simulink model "ReactorDistillation_scenario2_ratioV"  (R2024a)
settings: Solver=VariableStepAuto  StartTime=0.0  StopTime=1200  RelTol=1e-3
libraries: slpidlib x4
settings Model: Creator=tmlouw  LastModifiedBy=tmlouw

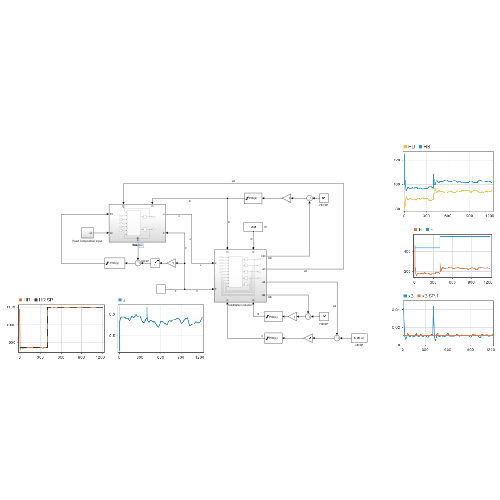
[thumbnail: Simulink's stored preview of the top-level diagram]
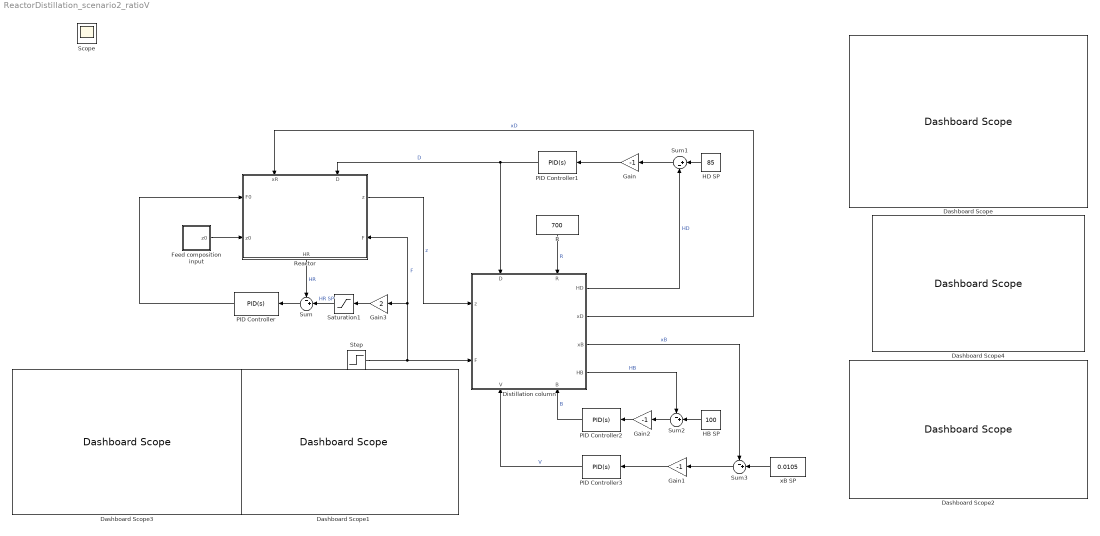
== system ReactorDistillation_scenario2_ratioV ==
  Dashboard Scope{,1,3..4} (4 alike) : DashboardScope
  Dashboard Scope2 : DashboardScope  Ymin=0  Ymax=0.05  ScaleAtStop=off
  Distillation column : Subsystem
      settings: PortSchema="{\"entries\":[{\"content\":{\"sides\":[{\"content\":{\"connectorIds\":[\"In1\",\"In2\"]},\"type\":\"ConnectorPlacement.EquallySpacedRectSide\",\"uuid\":\"ab420837-8800-483a-94a8-8143737a47c2\"},{\"content\":{\"connectorIds\":[\"Out1\",\"Out2\",\"Out3\",\"Out4\"],\"side\":\"RIGHT\"},\"type\":\"ConnectorPlacement.EquallySpacedRectSide\",\"uuid\":\"9920b73b-e391-416a-a827-f17b334a8e6d\"},{\"content\":{\"connectorIds\":[\"In3\",\"In4\"],\"side\":\"TOP\"},\"type\":\"ConnectorPlacement.EquallySpacedRectSide\",\"uuid\":\"f76ae38a-6a7c-4206-be40-6de8ba6ae5dc\"},{\"content\":{\"connectorIds\":[\"In5\",\"In6\"],\"side\":\"BOTTOM\"},\"type\":\"ConnectorPlacement.EquallySpacedRectSide\",\"uuid\":\"fa4d76dd-125e-48cb-976d-db25120835fd\"}]},\"type\":\"ConnectorPlacement.EquallySpacedConnector\",\"uuid\":\"aba5cf7b-c109-4372-afa3-985106281a24\"}],\"packageUris\":[\"http://schema.mathworks.com/mf0/Connector/R2020b\"],\"version\":\"1.0\"}"
  Feed composition input : Subsystem
  Gain : Gain  Gain=-1
  Gain1 : Gain  Gain=-1
  Gain2 : Gain  Gain=-1
  Gain3 : Gain  Gain=2
  HB SP : Constant  Value=100
  HD SP : Constant  Value=85
  PID Controller : slpidlib/PID Controller  Controller=PID  Form=Parallel  TimeDomain=Continuous-time  UseExternalTs=off  SampleTime=-1  IntegratorMethod=Forward Euler  FilterMethod=Forward Euler  ControllerParametersSource=internal  P=10  I=1  UseKiTs=off  D=0  UseExternalDerivativeSource=off  N=100  UseFilter=on  TunerSelectOption=Transfer Function Based (PID Tuner App)  InitialConditionSource=internal  InitialConditionForIntegrator=210  InitialConditionForFilter=0  DifferentiatorICPrevScaledInput=0  ExternalReset=none  TrackingMode=off  Kt=1  LimitOutput=on  SatLimitsSource=internal  UpperSaturationLimit=inf  LowerSaturationLimit=0  LinearizeAsGain=on  AntiWindupMode=none  Kb=1  LimitIntegrator=off  UpperIntegratorSaturationLimit=inf  LowerIntegratorSaturationLimit=-inf  POutMin=[]  POutMax=[]  IOutMin=[]  IOutMax=[]  DOutMin=[]  DOutMax=[]  NOutMin=[]  NOutMax=[]  SumOutMin=[]  SumOutMax=[]  SaturationOutMin=[]  SaturationOutMax=[]  PParamMin=[]  PParamMax=[]  IParamMin=[]  IParamMax=[]  DParamMin=[]  DParamMax=[]  NParamMin=[]  NParamMax=[]  KbParamMin=[]  KbParamMax=[]  KtParamMin=[]  KtParamMax=[]  KbOutMin=[]  KbOutMax=[]  KtOutMin=[]  KtOutMax=[]  IntegratorOutMin=[]  IntegratorOutMax=[]  FilterOutMin=[]  FilterOutMax=[]  SumI1OutMin=[]  SumI1OutMax=[]  SumI2OutMin=[]  SumI2OutMax=[]  SumI3OutMin=[]  SumI3OutMax=[]  SumI4OutMin=[]  SumI4OutMax=[]  SumDOutMin=[]  SumDOutMax=[]  DifferentiatorOutMin=[]  DifferentiatorOutMax=[]  FilterDiffOutCoefMin=[]  FilterDiffOutCoefMax=[]  ReciprocalOutMin=[]  ReciprocalOutMax=[]  SumDenOutMin=[]  SumDenOutMax=[]  SumNumOutMin=[]  SumNumOutMax=[]  DivideOutMin=[]  DivideOutMax=[]  UdiffTsProdOutMin=[]  UdiffTsProdOutMax=[]  NTsProdOutMin=[]  NTsProdOutMax=[]  UintegralTsProdOutMin=[]  UintegralTsProdOutMax=[]  UngainTsProdOutMin=[]  UngainTsProdOutMax=[]  ClampingZeroOutDataTypeStr=Inherit: Inherit via back propagation  ClampingZeroOutMin=[]  ClampingZeroOutMax=[]  FilterDenConstantOutDataTypeStr=Inherit: Inherit via back propagation  FilterDenConstantOutMin=[]  FilterDenConstantOutMax=[]  PCopyOutDataTypeStr=Inherit: Inherit via back propagation  PCopyOutMin=[]  PCopyOutMax=[]  NCopyOutDataTypeStr=Inherit: Inherit via back propagation  NCopyOutMin=[]  NCopyOutMax=[]  IntegratorContinuousStateAttributes=''  IntegratorStateMustResolveToSignalObject=off  IntegratorRTWStateStorageClass=Auto  FilterContinuousStateAttributes=''  FilterStateMustResolveToSignalObject=off  FilterRTWStateStorageClass=Auto  ParallelPVariant=InternalParameters  IdealPVariant=Disabled  IVariant=InternalParameters  DVariant=InternalParameters  IntegratorVariant=Continuous  SatVariant=Enabled  AWVariant=Passthrough  PCopyVariant=Disabled  TRVariant=Disabled  FdbkBlocksVariant=Forward  IdealPFdbkVariant=Disabled  SatFdbkVariant=Disabled  DerivativeFilterVariant=ContFilter  NVariant=InternalParameters  NCopyVariant=Disabled  FilterICVariant=InternalICsFilter  IntegratorICVariant=InternalICs  ExternalResetVariant=Disabled  TRSumVariant=Passthrough  SumFdbkVariant=Disabled  SumVariant=Sum_PID  TsampFilterVariant=InternalTs  TsampNgainVariant=Passthrough  TsampIntegralVariant=Disabled_SignalSpec  ExternalSaturationOutDataTypeStr=Inherit: Same as second input  DerivativeSourceVariant=ErrorSignal
  PID Controller1 : slpidlib/PID Controller  Controller=PID  Form=Parallel  TimeDomain=Continuous-time  UseExternalTs=off  SampleTime=-1  IntegratorMethod=Forward Euler  FilterMethod=Forward Euler  ControllerParametersSource=internal  P=10  I=0  UseKiTs=off  D=0  UseExternalDerivativeSource=off  N=100  UseFilter=on  TunerSelectOption=Transfer Function Based (PID Tuner App)  InitialConditionSource=internal  InitialConditionForIntegrator=225  InitialConditionForFilter=0  DifferentiatorICPrevScaledInput=0  ExternalReset=none  TrackingMode=off  Kt=1  LimitOutput=on  SatLimitsSource=internal  UpperSaturationLimit=inf  LowerSaturationLimit=0  LinearizeAsGain=on  AntiWindupMode=none  Kb=1  LimitIntegrator=off  UpperIntegratorSaturationLimit=inf  LowerIntegratorSaturationLimit=-inf  POutMin=[]  POutMax=[]  IOutMin=[]  IOutMax=[]  DOutMin=[]  DOutMax=[]  NOutMin=[]  NOutMax=[]  SumOutMin=[]  SumOutMax=[]  SaturationOutMin=[]  SaturationOutMax=[]  PParamMin=[]  PParamMax=[]  IParamMin=[]  IParamMax=[]  DParamMin=[]  DParamMax=[]  NParamMin=[]  NParamMax=[]  KbParamMin=[]  KbParamMax=[]  KtParamMin=[]  KtParamMax=[]  KbOutMin=[]  KbOutMax=[]  KtOutMin=[]  KtOutMax=[]  IntegratorOutMin=[]  IntegratorOutMax=[]  FilterOutMin=[]  FilterOutMax=[]  SumI1OutMin=[]  SumI1OutMax=[]  SumI2OutMin=[]  SumI2OutMax=[]  SumI3OutMin=[]  SumI3OutMax=[]  SumI4OutMin=[]  SumI4OutMax=[]  SumDOutMin=[]  SumDOutMax=[]  DifferentiatorOutMin=[]  DifferentiatorOutMax=[]  FilterDiffOutCoefMin=[]  FilterDiffOutCoefMax=[]  ReciprocalOutMin=[]  ReciprocalOutMax=[]  SumDenOutMin=[]  SumDenOutMax=[]  SumNumOutMin=[]  SumNumOutMax=[]  DivideOutMin=[]  DivideOutMax=[]  UdiffTsProdOutMin=[]  UdiffTsProdOutMax=[]  NTsProdOutMin=[]  NTsProdOutMax=[]  UintegralTsProdOutMin=[]  UintegralTsProdOutMax=[]  UngainTsProdOutMin=[]  UngainTsProdOutMax=[]  ClampingZeroOutDataTypeStr=Inherit: Inherit via back propagation  ClampingZeroOutMin=[]  ClampingZeroOutMax=[]  FilterDenConstantOutDataTypeStr=Inherit: Inherit via back propagation  FilterDenConstantOutMin=[]  FilterDenConstantOutMax=[]  PCopyOutDataTypeStr=Inherit: Inherit via back propagation  PCopyOutMin=[]  PCopyOutMax=[]  NCopyOutDataTypeStr=Inherit: Inherit via back propagation  NCopyOutMin=[]  NCopyOutMax=[]  IntegratorContinuousStateAttributes=''  IntegratorStateMustResolveToSignalObject=off  IntegratorRTWStateStorageClass=Auto  FilterContinuousStateAttributes=''  FilterStateMustResolveToSignalObject=off  FilterRTWStateStorageClass=Auto  ParallelPVariant=InternalParameters  IdealPVariant=Disabled  IVariant=InternalParameters  DVariant=InternalParameters  IntegratorVariant=Continuous  SatVariant=Enabled  AWVariant=Passthrough  PCopyVariant=Disabled  TRVariant=Disabled  FdbkBlocksVariant=Forward  IdealPFdbkVariant=Disabled  SatFdbkVariant=Disabled  DerivativeFilterVariant=ContFilter  NVariant=InternalParameters  NCopyVariant=Disabled  FilterICVariant=InternalICsFilter  IntegratorICVariant=InternalICs  ExternalResetVariant=Disabled  TRSumVariant=Passthrough  SumFdbkVariant=Disabled  SumVariant=Sum_PID  TsampFilterVariant=InternalTs  TsampNgainVariant=Passthrough  TsampIntegralVariant=Disabled_SignalSpec  ExternalSaturationOutDataTypeStr=Inherit: Same as second input  DerivativeSourceVariant=ErrorSignal
  PID Controller2 : slpidlib/PID Controller  Controller=PID  Form=Parallel  TimeDomain=Continuous-time  UseExternalTs=off  SampleTime=-1  IntegratorMethod=Forward Euler  FilterMethod=Forward Euler  ControllerParametersSource=internal  P=10  I=0  UseKiTs=off  D=0  UseExternalDerivativeSource=off  N=100  UseFilter=on  TunerSelectOption=Transfer Function Based (PID Tuner App)  InitialConditionSource=internal  InitialConditionForIntegrator=210  InitialConditionForFilter=0  DifferentiatorICPrevScaledInput=0  ExternalReset=none  TrackingMode=off  Kt=1  LimitOutput=on  SatLimitsSource=internal  UpperSaturationLimit=inf  LowerSaturationLimit=0  LinearizeAsGain=on  AntiWindupMode=none  Kb=1  LimitIntegrator=off  UpperIntegratorSaturationLimit=inf  LowerIntegratorSaturationLimit=-inf  POutMin=[]  POutMax=[]  IOutMin=[]  IOutMax=[]  DOutMin=[]  DOutMax=[]  NOutMin=[]  NOutMax=[]  SumOutMin=[]  SumOutMax=[]  SaturationOutMin=[]  SaturationOutMax=[]  PParamMin=[]  PParamMax=[]  IParamMin=[]  IParamMax=[]  DParamMin=[]  DParamMax=[]  NParamMin=[]  NParamMax=[]  KbParamMin=[]  KbParamMax=[]  KtParamMin=[]  KtParamMax=[]  KbOutMin=[]  KbOutMax=[]  KtOutMin=[]  KtOutMax=[]  IntegratorOutMin=[]  IntegratorOutMax=[]  FilterOutMin=[]  FilterOutMax=[]  SumI1OutMin=[]  SumI1OutMax=[]  SumI2OutMin=[]  SumI2OutMax=[]  SumI3OutMin=[]  SumI3OutMax=[]  SumI4OutMin=[]  SumI4OutMax=[]  SumDOutMin=[]  SumDOutMax=[]  DifferentiatorOutMin=[]  DifferentiatorOutMax=[]  FilterDiffOutCoefMin=[]  FilterDiffOutCoefMax=[]  ReciprocalOutMin=[]  ReciprocalOutMax=[]  SumDenOutMin=[]  SumDenOutMax=[]  SumNumOutMin=[]  SumNumOutMax=[]  DivideOutMin=[]  DivideOutMax=[]  UdiffTsProdOutMin=[]  UdiffTsProdOutMax=[]  NTsProdOutMin=[]  NTsProdOutMax=[]  UintegralTsProdOutMin=[]  UintegralTsProdOutMax=[]  UngainTsProdOutMin=[]  UngainTsProdOutMax=[]  ClampingZeroOutDataTypeStr=Inherit: Inherit via back propagation  ClampingZeroOutMin=[]  ClampingZeroOutMax=[]  FilterDenConstantOutDataTypeStr=Inherit: Inherit via back propagation  FilterDenConstantOutMin=[]  FilterDenConstantOutMax=[]  PCopyOutDataTypeStr=Inherit: Inherit via back propagation  PCopyOutMin=[]  PCopyOutMax=[]  NCopyOutDataTypeStr=Inherit: Inherit via back propagation  NCopyOutMin=[]  NCopyOutMax=[]  IntegratorContinuousStateAttributes=''  IntegratorStateMustResolveToSignalObject=off  IntegratorRTWStateStorageClass=Auto  FilterContinuousStateAttributes=''  FilterStateMustResolveToSignalObject=off  FilterRTWStateStorageClass=Auto  ParallelPVariant=InternalParameters  IdealPVariant=Disabled  IVariant=InternalParameters  DVariant=InternalParameters  IntegratorVariant=Continuous  SatVariant=Enabled  AWVariant=Passthrough  PCopyVariant=Disabled  TRVariant=Disabled  FdbkBlocksVariant=Forward  IdealPFdbkVariant=Disabled  SatFdbkVariant=Disabled  DerivativeFilterVariant=ContFilter  NVariant=InternalParameters  NCopyVariant=Disabled  FilterICVariant=InternalICsFilter  IntegratorICVariant=InternalICs  ExternalResetVariant=Disabled  TRSumVariant=Passthrough  SumFdbkVariant=Disabled  SumVariant=Sum_PID  TsampFilterVariant=InternalTs  TsampNgainVariant=Passthrough  TsampIntegralVariant=Disabled_SignalSpec  ExternalSaturationOutDataTypeStr=Inherit: Same as second input  DerivativeSourceVariant=ErrorSignal
  PID Controller3 : slpidlib/PID Controller  Controller=PID  Form=Parallel  TimeDomain=Continuous-time  UseExternalTs=off  SampleTime=-1  IntegratorMethod=Forward Euler  FilterMethod=Forward Euler  ControllerParametersSource=internal  P=1000  I=300  UseKiTs=off  D=0  UseExternalDerivativeSource=off  N=100  UseFilter=on  TunerSelectOption=Transfer Function Based (PID Tuner App)  InitialConditionSource=internal  InitialConditionForIntegrator=725  InitialConditionForFilter=0  DifferentiatorICPrevScaledInput=0  ExternalReset=none  TrackingMode=off  Kt=1  LimitOutput=on  SatLimitsSource=internal  UpperSaturationLimit=inf  LowerSaturationLimit=0  LinearizeAsGain=on  AntiWindupMode=none  Kb=1  LimitIntegrator=off  UpperIntegratorSaturationLimit=inf  LowerIntegratorSaturationLimit=-inf  POutMin=[]  POutMax=[]  IOutMin=[]  IOutMax=[]  DOutMin=[]  DOutMax=[]  NOutMin=[]  NOutMax=[]  SumOutMin=[]  SumOutMax=[]  SaturationOutMin=[]  SaturationOutMax=[]  PParamMin=[]  PParamMax=[]  IParamMin=[]  IParamMax=[]  DParamMin=[]  DParamMax=[]  NParamMin=[]  NParamMax=[]  KbParamMin=[]  KbParamMax=[]  KtParamMin=[]  KtParamMax=[]  KbOutMin=[]  KbOutMax=[]  KtOutMin=[]  KtOutMax=[]  IntegratorOutMin=[]  IntegratorOutMax=[]  FilterOutMin=[]  FilterOutMax=[]  SumI1OutMin=[]  SumI1OutMax=[]  SumI2OutMin=[]  SumI2OutMax=[]  SumI3OutMin=[]  SumI3OutMax=[]  SumI4OutMin=[]  SumI4OutMax=[]  SumDOutMin=[]  SumDOutMax=[]  DifferentiatorOutMin=[]  DifferentiatorOutMax=[]  FilterDiffOutCoefMin=[]  FilterDiffOutCoefMax=[]  ReciprocalOutMin=[]  ReciprocalOutMax=[]  SumDenOutMin=[]  SumDenOutMax=[]  SumNumOutMin=[]  SumNumOutMax=[]  DivideOutMin=[]  DivideOutMax=[]  UdiffTsProdOutMin=[]  UdiffTsProdOutMax=[]  NTsProdOutMin=[]  NTsProdOutMax=[]  UintegralTsProdOutMin=[]  UintegralTsProdOutMax=[]  UngainTsProdOutMin=[]  UngainTsProdOutMax=[]  ClampingZeroOutDataTypeStr=Inherit: Inherit via back propagation  ClampingZeroOutMin=[]  ClampingZeroOutMax=[]  FilterDenConstantOutDataTypeStr=Inherit: Inherit via back propagation  FilterDenConstantOutMin=[]  FilterDenConstantOutMax=[]  PCopyOutDataTypeStr=Inherit: Inherit via back propagation  PCopyOutMin=[]  PCopyOutMax=[]  NCopyOutDataTypeStr=Inherit: Inherit via back propagation  NCopyOutMin=[]  NCopyOutMax=[]  IntegratorContinuousStateAttributes=''  IntegratorStateMustResolveToSignalObject=off  IntegratorRTWStateStorageClass=Auto  FilterContinuousStateAttributes=''  FilterStateMustResolveToSignalObject=off  FilterRTWStateStorageClass=Auto  ParallelPVariant=InternalParameters  IdealPVariant=Disabled  IVariant=InternalParameters  DVariant=InternalParameters  IntegratorVariant=Continuous  SatVariant=Enabled  AWVariant=Passthrough  PCopyVariant=Disabled  TRVariant=Disabled  FdbkBlocksVariant=Forward  IdealPFdbkVariant=Disabled  SatFdbkVariant=Disabled  DerivativeFilterVariant=ContFilter  NVariant=InternalParameters  NCopyVariant=Disabled  FilterICVariant=InternalICsFilter  IntegratorICVariant=InternalICs  ExternalResetVariant=Disabled  TRSumVariant=Passthrough  SumFdbkVariant=Disabled  SumVariant=Sum_PID  TsampFilterVariant=InternalTs  TsampNgainVariant=Passthrough  TsampIntegralVariant=Disabled_SignalSpec  ExternalSaturationOutDataTypeStr=Inherit: Same as second input  DerivativeSourceVariant=ErrorSignal
  R : Constant  Value=700
  Reactor : Subsystem
      settings: PortSchema="{\"entries\":[{\"content\":{\"sides\":[{\"content\":{\"connectorIds\":[\"In1\",\"In2\"]},\"type\":\"ConnectorPlacement.EquallySpacedRectSide\",\"uuid\":\"b3a1644d-c0d9-45f7-9186-664ea9b1d498\"},{\"content\":{\"connectorIds\":[\"Out1\",\"In5\"],\"side\":\"RIGHT\"},\"type\":\"ConnectorPlacement.EquallySpacedRectSide\",\"uuid\":\"a66bb60f-7391-4359-960b-fc3938d0b523\"},{\"content\":{\"connectorIds\":[\"In3\",\"In4\"],\"side\":\"TOP\"},\"type\":\"ConnectorPlacement.EquallySpacedRectSide\",\"uuid\":\"83491796-fd53-421c-9b3f-2cf79eed5869\"},{\"content\":{\"connectorIds\":[\"Out2\"],\"side\":\"BOTTOM\"},\"type\":\"ConnectorPlacement.EquallySpacedRectSide\",\"uuid\":\"6ef939f5-44e6-4bb1-b3ee-0927c318fc00\"}]},\"type\":\"ConnectorPlacement.EquallySpacedConnector\",\"uuid\":\"7cecb2e0-65e2-445b-9e5a-a984b0a4124e\"}],\"packageUris\":[\"http://schema.mathworks.com/mf0/Connector/R2020b\"],\"version\":\"1.0\"}"
  Saturation1 : Saturate  UpperLimit=1400  LowerLimit=100
  Step : Step  Time=400  Before=435  After=550  SampleTime=0
  Sum : Sum  Inputs=-+|
  Sum1 : Sum  Inputs=|+-
  Sum2 : Sum  Inputs=-+|
  Sum3 : Sum  Inputs=-+|
  xB SP : Constant  Value=0.0105
  Scope : Scope
  wires:
  PID Controller1/1 -> Distillation column/3(D), Reactor/4(D)  "D"
  Step/1 -> Gain3/1, Reactor/5(F), Distillation column/2(F)  "F"
  R/1 -> Distillation column/4(R)  "R"
  Reactor/1(z) -> Distillation column/1(z)  "z"
  Reactor/2(HR) -> Sum/1  "HR"
  Distillation column/3(xB) -> Sum3/1  "xB"
  Distillation column/2(xD) -> Reactor/3(xR)  "xD"
  PID Controller2/1 -> Distillation column/6(B)  "B"
  PID Controller/1 -> Reactor/1(F0)
  Feed composition input/1(z0) -> Reactor/2(z0)
  Distillation column/1(HD) -> Sum1/2  "HD"
  Distillation column/4(HB) -> Sum2/1  "HB"
  Sum/1 -> PID Controller/1
  HD SP/1 -> Sum1/1
  Sum1/1 -> Gain/1
  Gain/1 -> PID Controller1/1
  xB SP/1 -> Sum3/2
  Sum3/1 -> Gain1/1
  Gain1/1 -> PID Controller3/1
  PID Controller3/1 -> Distillation column/5(V)  "V"
  Gain2/1 -> PID Controller2/1
  Sum2/1 -> Gain2/1
  HB SP/1 -> Sum2/2
  Gain3/1 -> Saturation1/1
  Saturation1/1 -> Sum/2  "HR SP"

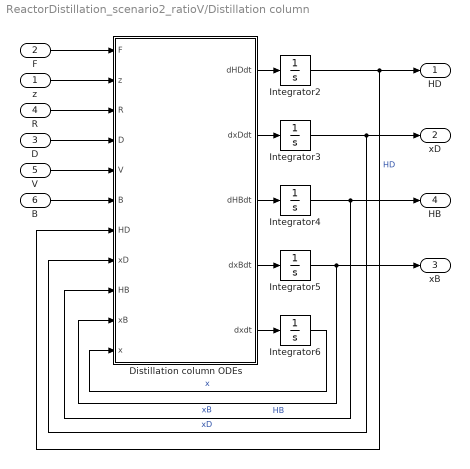
== system ReactorDistillation_scenario2_ratioV/Distillation column ==
  z : Inport
  F : Inport  Port=2
  D : Inport  Port=3
  R : Inport  Port=4
  V : Inport  Port=5
  B : Inport  Port=6
  Distillation column ODEs : MATLAB Function  TreatAsAtomicUnit=on
  Integrator2 : Integrator  InitialCondition=85  LimitOutput=on  LowerSaturationLimit=0
  Integrator3 : Integrator  InitialCondition=0.95  LimitOutput=on  UpperSaturationLimit=1  LowerSaturationLimit=0
  Integrator4 : Integrator  InitialCondition=124.738  LimitOutput=on  LowerSaturationLimit=0
  Integrator5 : Integrator  InitialCondition=0.0105  LimitOutput=on  UpperSaturationLimit=1  LowerSaturationLimit=0
  Integrator6 : Integrator  InitialCondition=0.5*ones(20,1)  LimitOutput=on  UpperSaturationLimit=ones(20,1)  LowerSaturationLimit=zeros(20,1)
  HD : Outport
  xD : Outport  Port=2
  xB : Outport  Port=3
  HB : Outport  Port=4
  wires:
  Integrator5/1 -> xB/1, Distillation column ODEs/10(xB)  "xB"
  Distillation column ODEs/3(dHBdt) -> Integrator4/1
  Distillation column ODEs/2(dxDdt) -> Integrator3/1
  Distillation column ODEs/1(dHDdt) -> Integrator2/1
  Integrator2/1 -> HD/1, Distillation column ODEs/7(HD)  "HD"
  Distillation column ODEs/4(dxBdt) -> Integrator5/1
  Distillation column ODEs/5(dxdt) -> Integrator6/1
  Integrator6/1 -> Distillation column ODEs/11(x)  "x"
  Integrator3/1 -> Distillation column ODEs/8(xD), xD/1  "xD"
  B/1 -> Distillation column ODEs/6(B)
  Integrator4/1 -> Distillation column ODEs/9(HB), HB/1  "HB"
  D/1 -> Distillation column ODEs/4(D)
  z/1 -> Distillation column ODEs/2(z)
  F/1 -> Distillation column ODEs/1(F)
  R/1 -> Distillation column ODEs/3(R)
  V/1 -> Distillation column ODEs/5(V)

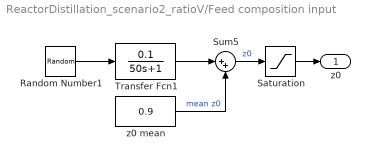
== system ReactorDistillation_scenario2_ratioV/Feed composition input ==
  Random Number1 : RandomNumber  SampleTime=30
  Saturation : Saturate  UpperLimit=1  LowerLimit=0.8
  Sum5 : Sum  Inputs=|++
  Transfer Fcn1 : TransferFcn  Numerator=[0.1]  Denominator=[50 1]
  z0 mean : Constant  Value=0.9
  z0 : Outport
  wires:
  Sum5/1 -> Saturation/1  "z0"
  z0 mean/1 -> Sum5/2  "mean z0"
  Saturation/1 -> z0/1
  Transfer Fcn1/1 -> Sum5/1
  Random Number1/1 -> Transfer Fcn1/1

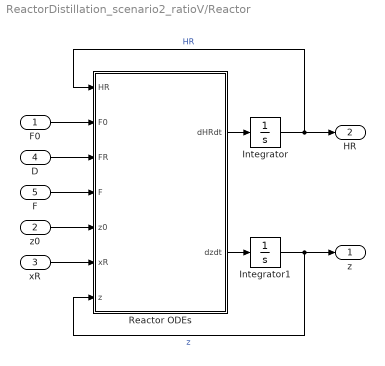
== system ReactorDistillation_scenario2_ratioV/Reactor ==
  F0 : Inport
  z0 : Inport  Port=2
  xR : Inport  Port=3
  D : Inport  Port=4
  F : Inport  Port=5
  Integrator : Integrator  InitialCondition=1088.622
  Integrator1 : Integrator  InitialCondition=0.5
  Reactor ODEs : MATLAB Function  TreatAsAtomicUnit=on
  z : Outport
  HR : Outport  Port=2
  wires:
  Reactor ODEs/1(dHRdt) -> Integrator/1
  Reactor ODEs/2(dzdt) -> Integrator1/1
  Integrator/1 -> HR/1, Reactor ODEs/1(HR)  "HR"
  D/1 -> Reactor ODEs/3(FR)
  F0/1 -> Reactor ODEs/2(F0)
  Integrator1/1 -> Reactor ODEs/7(z), z/1  "z"
  F/1 -> Reactor ODEs/4(F)
  xR/1 -> Reactor ODEs/6(xR)
  z0/1 -> Reactor ODEs/5(z0)

== matlab function ReactorDistillation_scenario2_ratioV/Distillation column/Distillation column ODEs ==
  data: F input; dHDdt output; z input; R input; D input; V input; B input; HD input; xD input; HB input; xB input; x input; dxDdt output; dHBdt output; dxBdt output; dxdt output
function [dHDdt, dxDdt, dHBdt, dxBdt, dxdt] = distillationODEs(F, z, R, D, V, B, HD, xD, HB, xB, x)
% Inputs:
% F: Feed flowrate (kmol/hr) [Reactor product flowrate in full model]
% z: Feed mol fraction (~) [Reactor product composition in full model]
% R: Reflux flowrate (kmol/hr)
% D: Distillate flowrate (kmol/hr)
% V: Reboil flowrate (kmol/hr)
% B: Bottoms flowrate (kmol/hr)
% HD: Condenser holdup (kmol)
% xD: Distillate mol fraction (~)
% HB: Reboiler holdup (kmol)
% xB: Bottoms mol fraction (~)
% x: vector corresponding to the liquid phase composition on each tray in the column,
%    i.e., x(1) is the liquid phase mol fraction on the bottom tray and 
%    x(20) is the liquid phase mol fraction on the top tray.

% Model parameters
nF = 12;          % Feed stage
HS = 124.738;     % kmol, Tray hold-up
alpha = 2;        % ~, relative volatility


dxdt = zeros(20,1); % Define derivative vector for tray compositions
L = R;              % Liquid flowrate above feed tray
Lb = L+F;           % Liquid flowrate below feed tray
y = alpha*x./(1 + x);    % Vapour phase mol fraction on each tray
yB = alpha*xB./(1 + xB); % Vapour phase mol fraction in the reboiler

% Condenser hold-up and composition
dHDdt = V - R - D;
dxDdt = V/HD*(y(20)-xD);

% Composition for all trays above the feed tray
i = nF+1 : 19;
dxdt(i)  = (  L*(x(i+1) - x(i) ) + V*(y(i-1) - y(i) )  )/HS;
dxdt(20) = (  L*(xD     - x(20)) + V*(y(19)  - y(20))  )/HS;

% Feed tray composition
dxdt(nF) = (  L*x(nF+1) - Lb*x(nF) + V*(y(nF-1) - y(nF)) + F*z  )/HS;

% Composition for all trays below the feed tray, (excl. bottom tray)
i = 2 : nF-1;
dxdt(i) = (  Lb*(x(i+1) - x(i)) + V*(y(i-1) - y(i))  )/HS;
dxdt(1) = (  Lb*(x(2)   - x(1)) + V*(yB     - y(1))  )/HS;

% Reboiler hold-up and composition
dHBdt = Lb - V - B;
dxBdt = (  Lb*(x(1) - xB) - V*(yB - xB)  )/HB;

== matlab function ReactorDistillation_scenario2_ratioV/Reactor/Reactor ODEs ==
  data: HR input; F0 input; FR input; dHRdt output; F input; z0 input; xR input; z input; dzdt output
function [dHRdt, dzdt] = reactorODEs(HR, F0, FR, F, z0, xR, z)
% Inputs:
% HR: Reactor holdup (kmol)
% F0: Feed flowrate (kmol/hr)
% FR: Recylce flowrate (kmol/hr) [Distillate flowrate in full model]
% F: Reactor product flowrate (kmol/hr)
% z0: Reactor feed mol fraction (~)
% xR: Recycle mol fraction (~) [Distillate mol fraction in full model]
% z: Reactor product mol fraction (~)

% Model parameters
kR = 0.33; % 1/hr, reaction rate constant

% Differential equations
dHRdt  = F0 + FR - F;
dzdt = F0/HR*(z0-z) + FR/HR*(xR-z) - kR*z;
